simulink model "trajectoryGenerator"  (R2022a)
settings: Solver=FixedStepDiscrete  StartTime=0.0  StopTime=8  FixedStep=0.001  RelTol=1e-3
values from neighbouring files (symbols this model uses):
  N = size(torqueData,1)    [coherenceTest.m]    (also in coherenceTestV2.m; fftTest.m = length(torque); firFilterParameter.m = Tout/Ts; firTest.m = Tout/Ts)
  Q0 = 0    [firFilterParameter.m]    (also in firTest.m)
  Ts = 0.001    [KalmanEstimator.m]    (also in firFilterParameter.m = samplingTime; firTest.m; leastSquare.m)
settings Model: Creator=kose  LastModifiedBy=kose

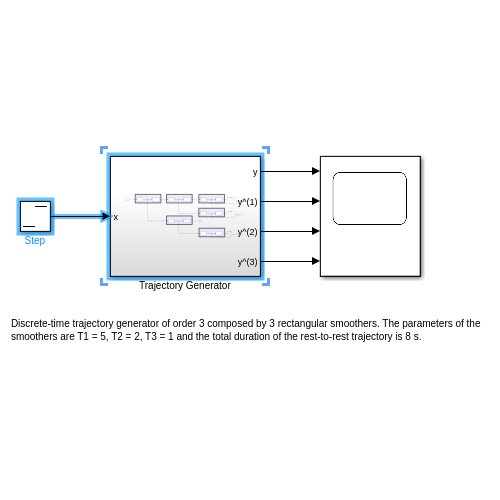
[thumbnail: Simulink's stored preview of the top-level diagram]
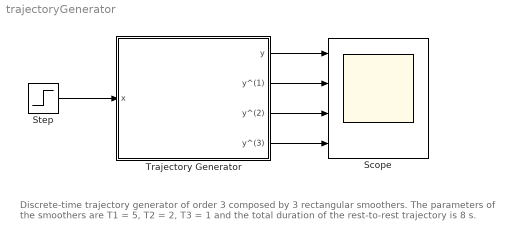
== system trajectoryGenerator ==
  note: Discrete-time trajectory generator of order 3 composed by 3 rectangular smoothers. The parameters of the smoothers are T1 = 5, T2 = 2, T3 = 1 and the total duration of the rest-to-rest trajectory is 8 s.
  Scope : Scope  NumInputPorts=4
  Step : Step  Time=0  After=100  SampleTime=0.001
  Trajectory Generator : Subsystem
  wires:
  Step/1 -> Trajectory Generator/1(x)
  Trajectory Generator/1(y) -> Scope/1
  Trajectory Generator/2(y^(1)) -> Scope/2
  Trajectory Generator/3(y^(2)) -> Scope/3
  Trajectory Generator/4(y^(3)) -> Scope/4

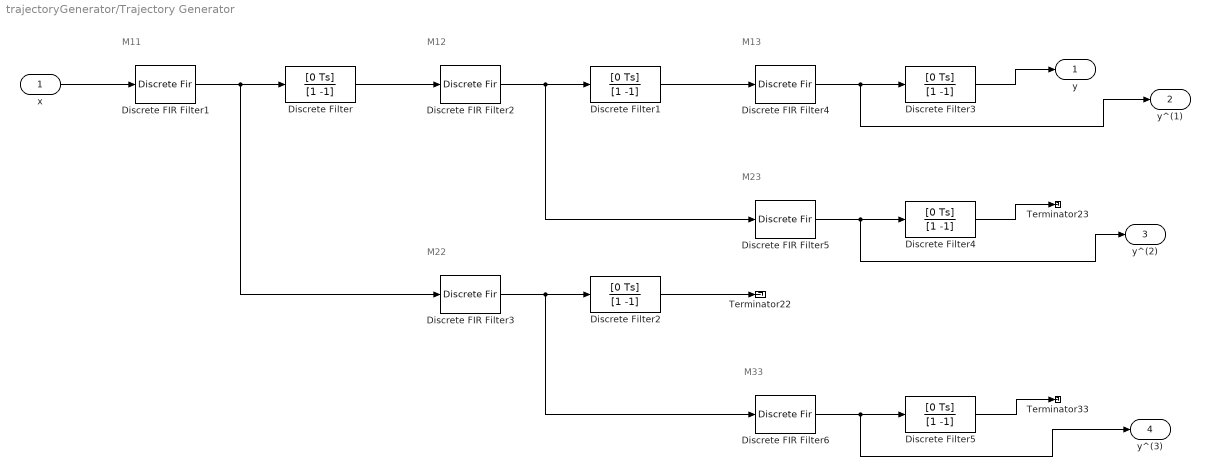
== system trajectoryGenerator/Trajectory Generator ==
  note: M33
  note: M23
  note: M13
  note: M22
  note: M12
  note: M11
  x : Inport
  Discrete FIR Filter1 : DiscreteFir  Coefficients=1/N(1)/Ts*[1 zeros(1,N(1)-1) -1]  InitialStates=Q0  SampleTime=Ts
  Discrete FIR Filter2 : DiscreteFir  Coefficients=1/N(2)/Ts*[1 zeros(1,N(2)-1) -1]  InitialStates=Q0  SampleTime=Ts
  Discrete FIR Filter3 : DiscreteFir  Coefficients=1/N(2)/Ts*[1 zeros(1,N(2)-1) -1]  InitialStates=Q0  SampleTime=Ts
  Discrete FIR Filter4 : DiscreteFir  Coefficients=1/N(3)/Ts*[1 zeros(1,N(3)-1) -1]  InitialStates=Q0  SampleTime=Ts
  Discrete FIR Filter5 : DiscreteFir  Coefficients=1/N(3)/Ts*[1 zeros(1,N(3)-1) -1]  InitialStates=Q0  SampleTime=Ts
  Discrete FIR Filter6 : DiscreteFir  Coefficients=1/N(3)/Ts*[1 zeros(1,N(3)-1) -1]  InitialStates=Q0  SampleTime=Ts
  Discrete Filter{,1..5} (6 alike) : DiscreteFilter  Numerator=[0 Ts]  Denominator=[1 -1]  InitialStates=Q0  SampleTime=Ts
  Terminator22 : Terminator
  Terminator23 : Terminator
  Terminator33 : Terminator
  y : Outport
  y^(1) : Outport  Port=2
  y^(2) : Outport  Port=3
  y^(3) : Outport  Port=4
  wires:
  Discrete Filter2/1 -> Terminator22/1
  Discrete Filter4/1 -> Terminator23/1
  Discrete Filter5/1 -> Terminator33/1
  Discrete Filter3/1 -> y/1
  Discrete FIR Filter4/1 -> y^(1)/1, Discrete Filter3/1
  Discrete FIR Filter5/1 -> y^(2)/1, Discrete Filter4/1
  Discrete FIR Filter6/1 -> y^(3)/1, Discrete Filter5/1
  x/1 -> Discrete FIR Filter1/1
  Discrete Filter/1 -> Discrete FIR Filter2/1
  Discrete FIR Filter1/1 -> Discrete FIR Filter3/1, Discrete Filter/1
  Discrete Filter1/1 -> Discrete FIR Filter4/1
  Discrete FIR Filter2/1 -> Discrete FIR Filter5/1, Discrete Filter1/1
  Discrete FIR Filter3/1 -> Discrete FIR Filter6/1, Discrete Filter2/1
